simulink library "LeverArm"  (R2014b)
settings: Solver=ode45  StartTime=0.0  StopTime=10.0  RelTol=1e-3
undefined symbols (not defined in the file or in its folder): ConfParam
libraries: DivisionVectorScalar x1, Normalization x1
settings Model: Creator=Hp  LastModifiedBy=Hp

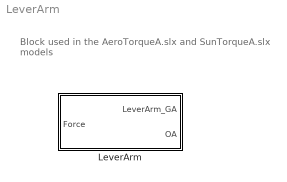
== system LeverArm ==
  note: Block used in the AeroTorqueA.slx
      | and SunTorqueA.slx models
  LeverArm : Subsystem

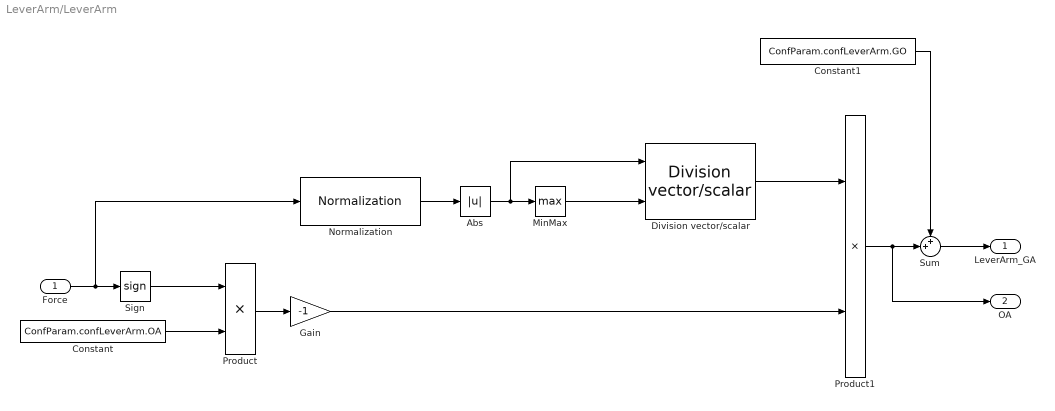
== system LeverArm/LeverArm ==
  Force : Inport
  Abs : Abs
  Constant : Constant  Value=ConfParam.confLeverArm.OA
  Constant1 : Constant  Value=ConfParam.confLeverArm.GO
  Division vector/scalar : DivisionVectorScalar/Division vector//scalar
  Gain : Gain  Gain=-1
  MinMax : MinMax  Function=max
  Normalization : Normalization/Normalization
  Product : Product
  Product1 : Product
  Sign : Signum
  Sum : Sum  Inputs=++|
  LeverArm_GA : Outport
  OA : Outport  Port=2
  wires:
  Constant/1 -> Product/2
  Sign/1 -> Product/1
  Gain/1 -> Product1/2
  Normalization/1 -> Abs/1
  Division vector/scalar/1 -> Product1/1
  Abs/1 -> Division vector/scalar/1, MinMax/1
  Product/1 -> Gain/1
  Force/1 -> Normalization/1, Sign/1
  Constant1/1 -> Sum/1
  Sum/1 -> LeverArm_GA/1
  MinMax/1 -> Division vector/scalar/2
  Product1/1 -> OA/1, Sum/2
